simulink model "PID_controller"  (R2024b)
settings: Solver=ode5  StartTime=0.0  StopTime=10  FixedStep=10e-06  RelTol=1e-3
undefined symbols (not defined in the file): DiscIntNeverNeededParam, index, K_vec, Nu, Nx, rpm2rads, T, u_bar_max
settings Model: Creator=Enrico  LastModifiedBy=farin
settings DataIOCC: ReturnWorkspaceOutputsName=out_black_box

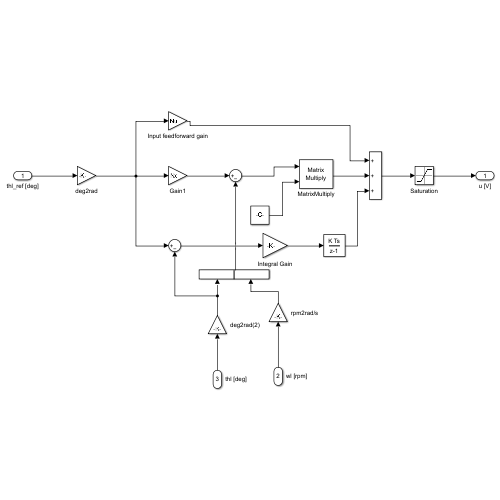
[thumbnail: Simulink's stored preview of the top-level diagram]
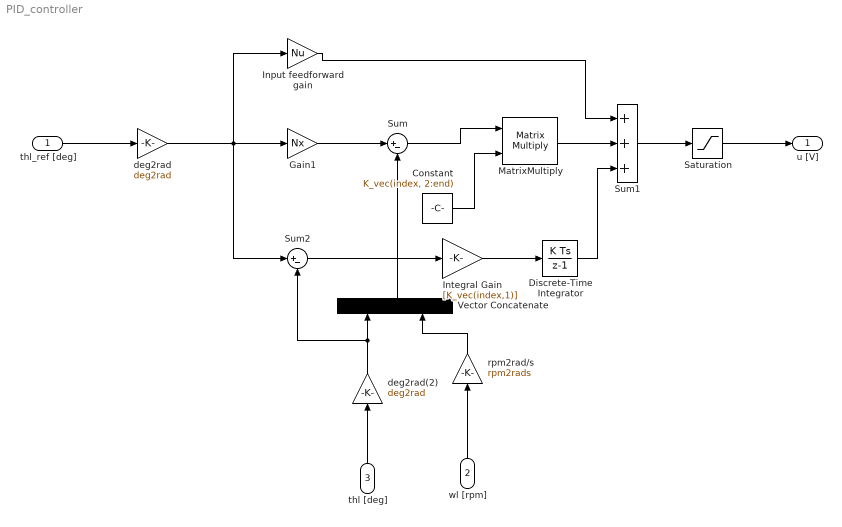
== system PID_controller ==
  thl_ref [deg] : Inport
  wl [rpm] : Inport  Port=2
  thl [deg] : Inport  Port=3
  Constant : Constant  Value=K_vec(index, 2:end)
  Discrete-Time Integrator : DiscreteIntegrator  SampleTime=T  ICPrevOutput=DiscIntNeverNeededParam  ICPrevScaledInput=DiscIntNeverNeededParam
  Gain1 : Gain  Gain=Nx
  Input feedforward gain : Gain  Gain=Nu
  Integral Gain : Gain  Gain=[K_vec(index,1)]
  MatrixMultiply : Product  Multiplication=Matrix(*)
  Saturation : Saturate  UpperLimit=u_bar_max  LowerLimit=-u_bar_max
  Sum : Sum  Inputs=|+-
  Sum1 : Sum  Inputs=+++
  Sum2 : Sum  Inputs=|+-
  Vector Concatenate : Concatenate
  deg2rad : Gain  Gain=deg2rad
  deg2rad(2) : Gain  Gain=deg2rad
  rpm2rad/s : Gain  Gain=rpm2rads
  u [V] : Outport
  wires:
  Gain1/1 -> Sum/1
  Discrete-Time Integrator/1 -> Sum1/3
  thl_ref [deg]/1 -> deg2rad/1
  Saturation/1 -> u [V]/1
  deg2rad(2)/1 -> Vector Concatenate/1, Sum2/2
  Sum/1 -> MatrixMultiply/1
  Input feedforward gain/1 -> Sum1/1
  Sum1/1 -> Saturation/1
  Integral Gain/1 -> Discrete-Time Integrator/1
  Constant/1 -> MatrixMultiply/2
  MatrixMultiply/1 -> Sum1/2
  thl [deg]/1 -> deg2rad(2)/1
  deg2rad/1 -> Gain1/1, Sum2/1, Input feedforward gain/1
  wl [rpm]/1 -> rpm2rad/s/1
  Vector Concatenate/1 -> Sum/2
  rpm2rad/s/1 -> Vector Concatenate/2
  Sum2/1 -> Integral Gain/1
